simulink model "Masse_MultirotorSimHinf"  (R2018b)
settings: Solver=VariableStepAuto  StartTime=0.0  StopTime=Simulation.T_END  MaxStep=Simulation.TS_MAX  RelTol=1e-3  EnableMultiTasking=on
PreLoadFcn:
  | % InitializeParameters;
undefined symbols (not defined in the file): Aero, armed, ctrl_state, INIT_PARAM_VECTOR, Initial, K_i, K_p, Motor, mpc_att_sp, mpc_ctrl_state, mpc_manual, mpc_pos_sp_triplet, mpc_vehicle_land_detected, mpc_vehicle_status, Simulation, SOF1, SOF2, Uav, Upsilon, v_att_sp, v_control_mode
libraries: simulink_extras x9, simulink x6, dspstat3 x1, Px4Library x1
(part 11 of 11)

== matlab function Masse_MultirotorSimHinf/Quadrotor Quaternion Model/Quaternion to Euler Angles/MATLAB Function ==
  data: quat input; eul output
function eul   = QuaternionToEuler( quat )
%QUATERNIONTOEULER Convert quaternion to euler angles
%   Based on PX4 Firmware code: https://github.com/PX4/Firmware
%   Written by:    J.X.J. Bannwarth, 2016/08/29
%   Last modified: J.X.J. Bannwarth, 2018/12/11

    eul = [ atan2(2.0 .* (quat(1) .* quat(2) + quat(3) .* quat(4)), ...
                1.0 - 2.0 .* (quat(2) .* quat(2) + quat(3) .* quat(3)));
	        asin(2.0 .* (quat(1) .* quat(3) - quat(4) .* quat(2)));
            atan2(2.0 .* (quat(1) .* quat(4) + quat(2) .* quat(3)), ...
                1.0 - 2.0 .* (quat(3) .* quat(3) + quat(4) .* quat(4))) ];
end

== matlab function Masse_MultirotorSimHinf/att_mixerInput/Quaternion to Euler Angles3/MATLAB Function ==
  data: quat input; eul output
function eul   = QuaternionToEuler( quat )
%QUATERNIONTOEULER Convert quaternion to euler angles
%   Based on PX4 Firmware code: https://github.com/PX4/Firmware
%   Written by:    J.X.J. Bannwarth, 2016/08/29
%   Last modified: J.X.J. Bannwarth, 2018/12/11

    eul = [ atan2(2.0 .* (quat(1) .* quat(2) + quat(3) .* quat(4)), ...
                1.0 - 2.0 .* (quat(2) .* quat(2) + quat(3) .* quat(3)));
	        asin(2.0 .* (quat(1) .* quat(3) - quat(4) .* quat(2)));
            atan2(2.0 .* (quat(1) .* quat(4) + quat(2) .* quat(3)), ...
                1.0 - 2.0 .* (quat(3) .* quat(3) + quat(4) .* quat(4))) ];
end
